simulink subsystem "feed_lin_sagittal_sub"  (R2022b)
settings: Solver=VariableStepAuto  StartTime=0.0  StopTime=10.0  RelTol=1e-3
libraries: dspsigops x1
settings Model: Creator=Edp  LastModifiedBy=gotta

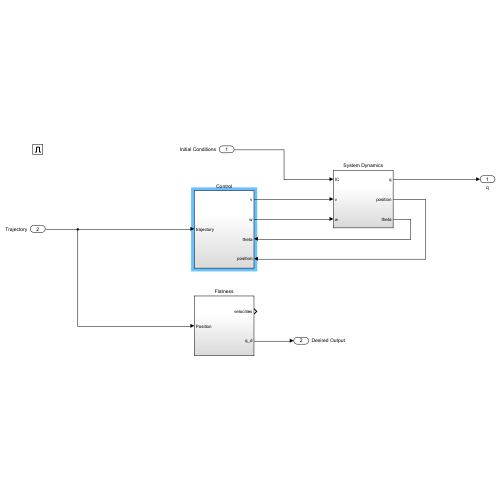
[thumbnail: Simulink's stored preview of the top-level diagram]
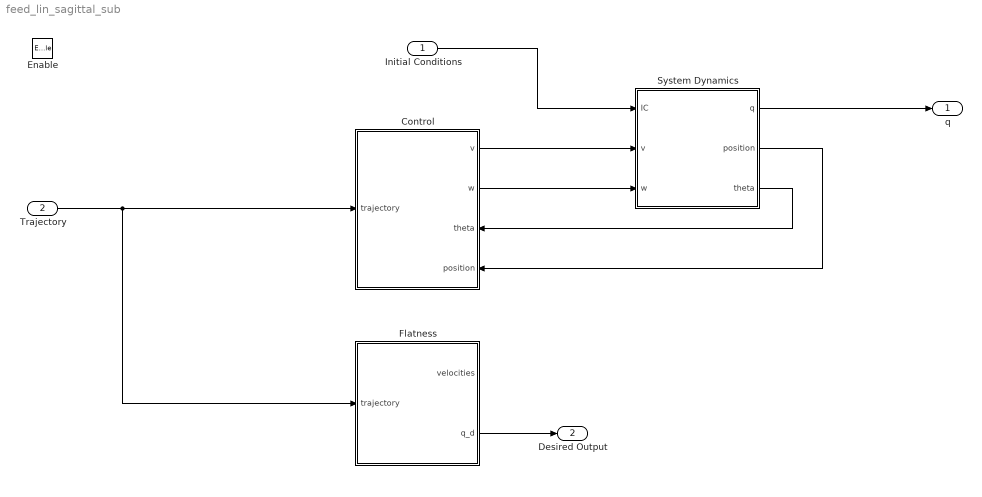
== system feed_lin_sagittal_sub ==
  Initial Conditions : Inport
  Trajectory : Inport  Port=2
  Enable : EnablePort
  Control : Subsystem
      settings: PortSchema="{\"entries\":[{\"content\":{\"sides\":[{\"content\":{\"connectorIds\":[\"In1\"]},\"type\":\"ConnectorPlacement.EquallySpacedRectSide\",\"uuid\":\"22e24f09-d087-4651-8454-98040f2d0294\"},{\"content\":{\"connectorIds\":[\"Out1\",\"Out2\",\"In2\",\"In3\"],\"side\":\"RIGHT\"},\"type\":\"ConnectorPlacement.EquallySpacedRectSide\",\"uuid\":\"e8a6b77f-aadd-4f7a-b37b-e349f2a70480\"},{\"content\":{\"connectorIds\":[],\"side\":\"TOP\"},\"type\":\"ConnectorPlacement.EquallySpacedRectSide\",\"uuid\":\"bc8ee2e9-946d-40b9-bedb-1332b8935ae7\"}]},\"type\":\"ConnectorPlacement.EquallySpacedConnector\",\"uuid\":\"a313642d-50c8-4734-aea6-49f18ad579f0\"}],\"packageUris\":[\"http://schema.mathworks.com/mf0/Connector/R2020b\"],\"version\":\"1.0\"}"
  Flatness : Subsystem
  System Dynamics : Subsystem
  q : Outport
  Desired Output : Outport  Port=2
  wires:
  Initial Conditions/1 -> System Dynamics/1(IC)
  System Dynamics/1(q) -> q/1
  System Dynamics/3(theta) -> Control/2(theta)
  Trajectory/1 -> Flatness/1(trajectory), Control/1(trajectory)
  Control/2(w) -> System Dynamics/3(w)
  Control/1(v) -> System Dynamics/2(v)
  Flatness/2(q_d) -> Desired Output/1
  System Dynamics/2(position) -> Control/3(position)

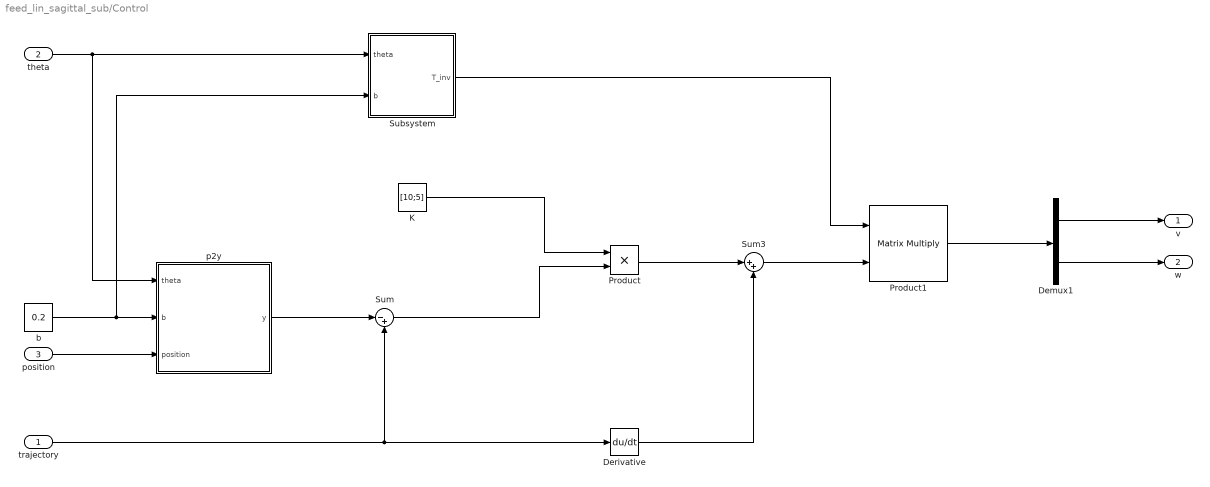
== system feed_lin_sagittal_sub/Control ==
  trajectory : Inport
  theta : Inport  Port=2
  position : Inport  Port=3
  Demux1 : Demux  Outputs=2
  Derivative : Derivative
  K : Constant  Value=[10;5]
  Product : Product
  Product1 : Product  Multiplication=Matrix(*)
  Subsystem : Subsystem
  Sum : Sum  Inputs=|-+
  Sum3 : Sum  Inputs=|++
  b : Constant  Value=0.2
  p2y : Subsystem
      settings: PortSchema="{\"entries\":[{\"content\":{\"sides\":[{\"content\":{\"connectorIds\":[\"Out1\"]},\"type\":\"ConnectorPlacement.EquallySpacedRectSide\",\"uuid\":\"22e24f09-d087-4651-8454-98040f2d0294\"},{\"content\":{\"connectorIds\":[\"In1\",\"In2\",\"In3\"],\"side\":\"RIGHT\"},\"type\":\"ConnectorPlacement.EquallySpacedRectSide\",\"uuid\":\"e8a6b77f-aadd-4f7a-b37b-e349f2a70480\"},{\"content\":{\"connectorIds\":[],\"side\":\"TOP\"},\"type\":\"ConnectorPlacement.EquallySpacedRectSide\",\"uuid\":\"bc8ee2e9-946d-40b9-bedb-1332b8935ae7\"}]},\"type\":\"ConnectorPlacement.EquallySpacedConnector\",\"uuid\":\"a313642d-50c8-4734-aea6-49f18ad579f0\"}],\"packageUris\":[\"http://schema.mathworks.com/mf0/Connector/R2020b\"],\"version\":\"1.0\"}"
  v : Outport
  w : Outport  Port=2
  wires:
  Subsystem/1(T_inv) -> Product1/1
  Sum/1 -> Product/2
  Demux1/2 -> w/1
  Product/1 -> Sum3/1
  Sum3/1 -> Product1/2
  Product1/1 -> Demux1/1
  K/1 -> Product/1
  theta/1 -> p2y/3(theta), Subsystem/1(theta)
  trajectory/1 -> Sum/2, Derivative/1
  Demux1/1 -> v/1
  Derivative/1 -> Sum3/2
  b/1 -> Subsystem/2(b), p2y/2(b)
  position/1 -> p2y/1(position)
  p2y/1(y) -> Sum/1

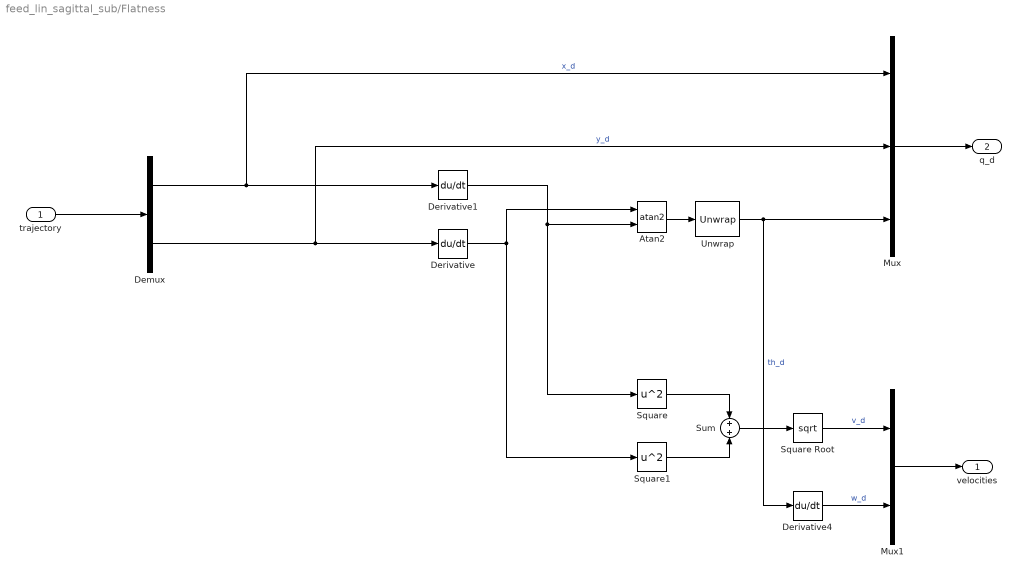
== system feed_lin_sagittal_sub/Flatness ==
  trajectory : Inport
  Atan2 : Trigonometry  Operator=atan2
  Demux : Demux  Outputs=2
  Derivative : Derivative
  Derivative1 : Derivative
  Derivative4 : Derivative
  Mux : Mux  Inputs=3
  Mux1 : Mux  Inputs=2
  Square : Math  Operator=square
  Square Root : Sqrt
  Square1 : Math  Operator=square
  Sum : Sum  Inputs=+|+
  Unwrap : dspsigops/Unwrap  tol=pi  running=off
  velocities : Outport
  q_d : Outport  Port=2
  wires:
  trajectory/1 -> Demux/1
  Unwrap/1 -> Mux/3, Derivative4/1  "th_d"
  Derivative4/1 -> Mux1/2  "w_d"
  Square Root/1 -> Mux1/1  "v_d"
  Mux1/1 -> velocities/1
  Sum/1 -> Square Root/1
  Square1/1 -> Sum/2
  Square/1 -> Sum/1
  Mux/1 -> q_d/1
  Demux/1 -> Derivative1/1, Mux/1  "x_d"
  Atan2/1 -> Unwrap/1
  Derivative1/1 -> Square/1, Atan2/2
  Demux/2 -> Derivative/1, Mux/2  "y_d"
  Derivative/1 -> Atan2/1, Square1/1

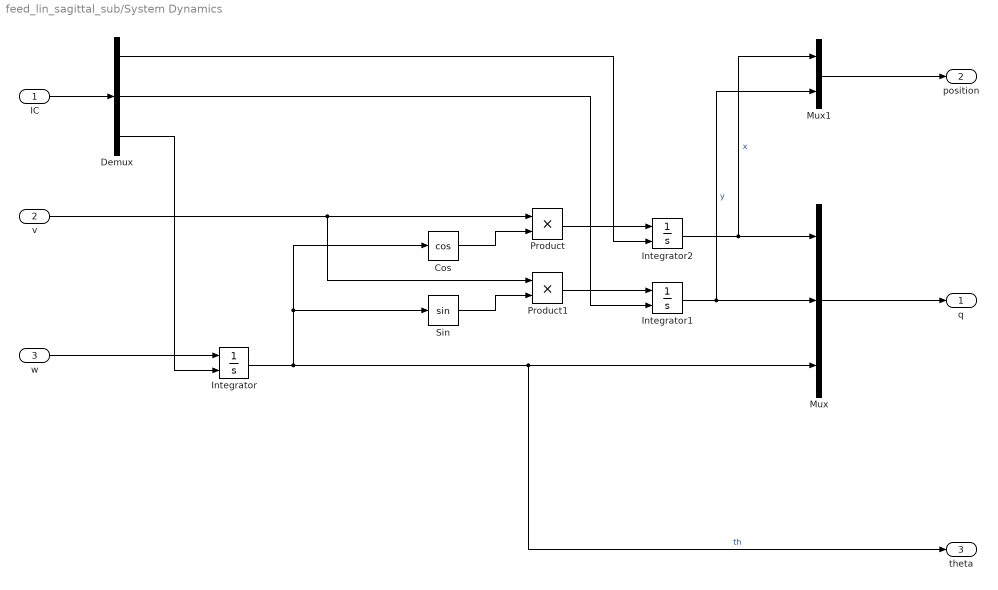
== system feed_lin_sagittal_sub/System Dynamics ==
  IC : Inport
  v : Inport  Port=2
  w : Inport  Port=3
  Cos : Trigonometry  Operator=cos
  Demux : Demux  Outputs=3
  Integrator : Integrator  InitialConditionSource=external
  Integrator1 : Integrator  InitialConditionSource=external
  Integrator2 : Integrator  InitialConditionSource=external
  Mux : Mux  Inputs=3
  Mux1 : Mux  Inputs=2
  Product : Product
  Product1 : Product
  Sin : Trigonometry
  q : Outport
  position : Outport  Port=2
  theta : Outport  Port=3
  wires:
  Demux/3 -> Integrator/2
  Demux/2 -> Integrator1/2
  Demux/1 -> Integrator2/2
  IC/1 -> Demux/1
  Cos/1 -> Product/2
  Integrator2/1 -> Mux/1, Mux1/1  "x"
  Sin/1 -> Product1/2
  Integrator1/1 -> Mux/2, Mux1/2  "y"
  Integrator/1 -> Cos/1, Sin/1, Mux/3, theta/1  "th"
  Product1/1 -> Integrator1/1
  Product/1 -> Integrator2/1
  v/1 -> Product/1, Product1/1
  w/1 -> Integrator/1
  Mux/1 -> q/1
  Mux1/1 -> position/1

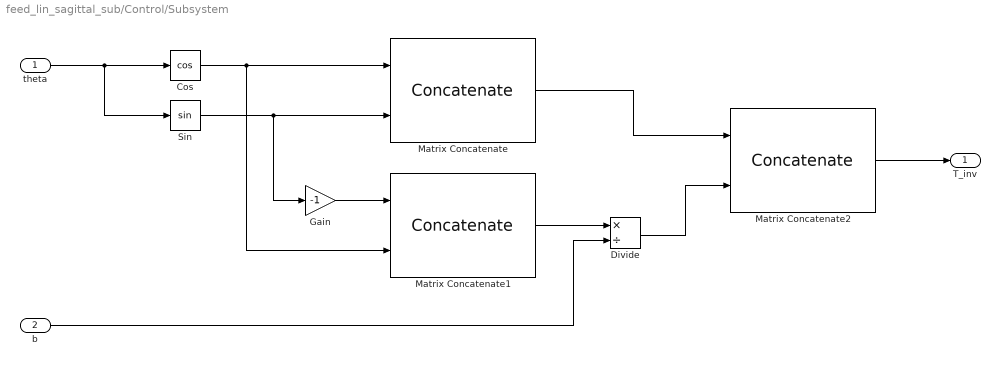
== system feed_lin_sagittal_sub/Control/Subsystem ==
  theta : Inport
  b : Inport  Port=2
  Cos : Trigonometry  Operator=cos
  Divide : Product  Inputs=*/
  Gain : Gain  Gain=-1
  Matrix Concatenate : Concatenate  Mode=Multidimensional array  ConcatenateDimension=2
  Matrix Concatenate1 : Concatenate  Mode=Multidimensional array  ConcatenateDimension=2
  Matrix Concatenate2 : Concatenate  Mode=Multidimensional array
  Sin : Trigonometry
  T_inv : Outport
  wires:
  theta/1 -> Sin/1, Cos/1
  Cos/1 -> Matrix Concatenate1/2, Matrix Concatenate/1
  Sin/1 -> Gain/1, Matrix Concatenate/2
  Gain/1 -> Matrix Concatenate1/1
  Matrix Concatenate1/1 -> Divide/1
  b/1 -> Divide/2
  Matrix Concatenate/1 -> Matrix Concatenate2/1
  Divide/1 -> Matrix Concatenate2/2
  Matrix Concatenate2/1 -> T_inv/1

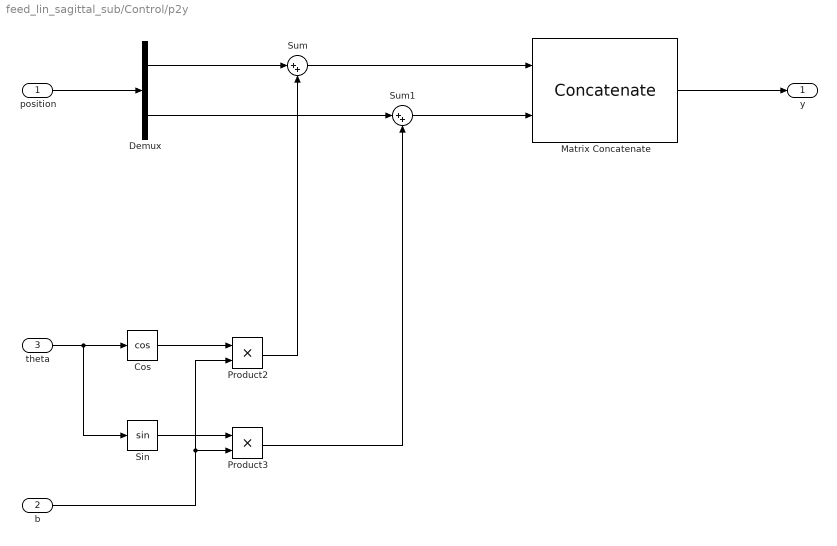
== system feed_lin_sagittal_sub/Control/p2y ==
  position : Inport
  b : Inport  Port=2
  theta : Inport  Port=3
  Cos : Trigonometry  Operator=cos
  Demux : Demux  Outputs=2
  Matrix Concatenate : Concatenate  Mode=Multidimensional array  ConcatenateDimension=2
  Product2 : Product
  Product3 : Product
  Sin : Trigonometry
  Sum : Sum  Inputs=|++
  Sum1 : Sum  Inputs=|++
  y : Outport
  wires:
  position/1 -> Demux/1
  theta/1 -> Sin/1, Cos/1
  Cos/1 -> Product2/1
  Sin/1 -> Product3/1
  Product2/1 -> Sum/2
  Product3/1 -> Sum1/2
  b/1 -> Product2/2, Product3/2
  Sum/1 -> Matrix Concatenate/1
  Sum1/1 -> Matrix Concatenate/2
  Matrix Concatenate/1 -> y/1
  Demux/1 -> Sum/1
  Demux/2 -> Sum1/1
